simulink model "generic_IVS"  (R2024a)
settings: Solver=FixedStepDiscrete  StartTime=0.0  StopTime=inf  FixedStep=0.001  RelTol=1e-3
undefined symbols (not defined in the file): do_waypoints_tail_shifted_2, pathXY, route1_waypoint, route1_waypoint_raw, route2_waypoint, route2_waypoint_raw, route3_waypoint, route3_waypoint_raw, waypoints2
libraries: CarMaker4SL x431, slpidlib x19, dspsigops x3, simulink x1
(part 7 of 15)

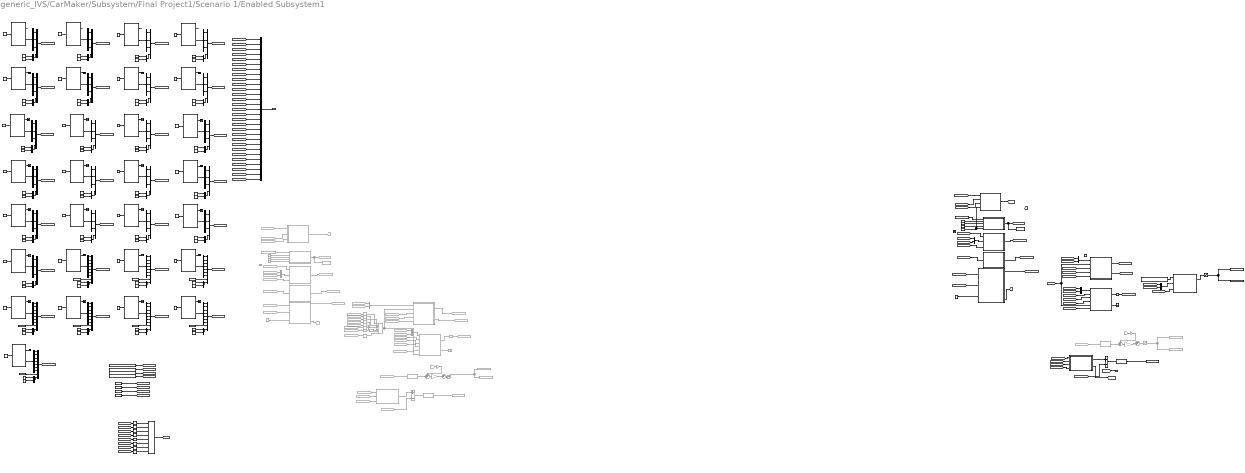
== system generic_IVS/CarMaker/Subsystem/Final Project1/Scenario 1/Enabled Subsystem1 ==
  note: Traffic Size
      | Length: 4.47
      | Width: 1.97
      | Height: 1.12
  note: 주행 개인
  note: Traffic Size
      | Length: 4.47
      | Width: 1.97
      | Height: 1.12
  note: Traffic Size
      | Length: 4.47
      | Width: 1.97
      | Height: 1.12
  note: Traffic Size
      | Length: 4.47
      | Width: 1.97
      | Height: 1.12
  note: Traffic Size
      | Length: 4.47
      | Width: 1.97
      | Height: 1.12
  note: Traffic Size
      | Length: 4.47
      | Width: 1.97
      | Height: 1.12
  note: Traffic Size
      | Length: 4.47
      | Width: 1.97
      | Height: 1.12
  note: Traffic Size
      | Length: 4.47
      | Width: 1.97
      | Height: 1.12
  note: 파킹 개인
  note: Traffic Size
      | Length: 4.47
      | Width: 1.97
      | Height: 1.12
  note: Traffic Size
      | Length: 4.47
      | Width: 1.97
      | Height: 1.12
  note: Traffic Size
      | Length: 4.47
      | Width: 1.97
      | Height: 1.12
  note: Traffic Size
      | Length: 4.47
      | Width: 1.97
      | Height: 1.12
  note: Traffic Size
      | Length: 4.47
      | Width: 1.97
      | Height: 1.12
  note: Traffic Size
      | Length: 4.47
      | Width: 1.97
      | Height: 1.12
  note: Traffic Size
      | Length: 4.47
      | Width: 1.97
      | Height: 1.12
  note: Traffic Size
      | Length: 4.47
      | Width: 1.97
      | Height: 1.12
  note: Traffic Size
      | Length: 4.47
      | Width: 1.97
      | Height: 1.12
  note: Traffic Size
      | Length: 4.47
      | Width: 1.97
      | Height: 1.12
  note: Traffic Size
      | Length: 4.47
      | Width: 1.97
      | Height: 1.12
  note: Traffic Size
      | Length: 4.47
      | Width: 1.97
      | Height: 1.12
  note: Traffic Size
      | Length: 4.47
      | Width: 1.97
      | Height: 1.12
  note: Modify !!
  note: Traffic Size
      | Length: 4.47
      | Width: 1.97
      | Height: 1.12
  note: Traffic Size
      | Length: 4.47
      | Width: 1.97
      | Height: 1.12
  note: Traffic Size
      | Length: 4.47
      | Width: 1.97
      | Height: 1.12
  note: Traffic Size
      | Length: 4.47
      | Width: 1.97
      | Height: 1.12
  note: Traffic Size
      | Length: 4.47
      | Width: 1.97
      | Height: 1.12
  note: Traffic Size
      | Length: 4.47
      | Width: 1.97
      | Height: 1.12
  note: 0: 파킹 경로, 1 주행, 2 파킹
  note: Traffic Size
      | Length: 4.47
      | Width: 1.97
      | Height: 1.12
  note: Average Filter
  note: Traffic Size
      | Length: 4.47
      | Width: 1.97
      | Height: 1.12
  note: Average Filter
  note: 0: 파킹 경로, 1 주행, 2 파킹
  note: Modify !!
  Enable : EnablePort
  Add : Sum  Inputs=+-
  Add1 : Sum  Commented=on  Inputs=+-
  Bus Selector{3..19,22,28..30} (21 alike) : BusSelector  OutputSignals=t_0 x,t_0 y,r_zyx z
  Bus Selector{20..21,23..27,31} (8 alike) : BusSelector  OutputSignals=t_0 x,t_0 y,v_0 x,v_0 y,a_0 x,a_0 y,r_zyx z
  Constant : Constant  Value=waypoints2
  Constant1 : Constant  Commented=on  Value=1565
  Constant10 : Constant  Commented=on
  Constant11 : Constant
  Constant110 : Constant  Value=do_waypoints_tail_shifted_2
  Constant111 : Constant  Value=1565
  Constant114 : Constant  Value=do_waypoints_tail_shifted_2
  Constant115 : Constant  Value=942
  Constant116 : Constant  Value=0
  Constant117 : Constant  Value=0
  Constant12 : Constant  Value=5
  Constant{13,16,19,21..22,26,29,32,35,39,42,46,48,52,55..56,59,61,65,69,72,74,79,82,85,87..88,92,96} (29 alike) : Constant  Value=4.47
  Constant{14,17,23..24,27,30,33,36..37,40,43,49..50,53,57,62..63,66..67,70,75..76,80,83,89..90,93..94,97} (29 alike) : Constant  Value=1.97
  Constant15 : Constant  Value=7
  Constant18 : Constant  Value=8
  Constant2 : Constant  Commented=on  Value=do_waypoints_tail_shifted_2
  Constant20 : Constant  Value=4
  Constant25 : Constant  Value=10
  Constant28 : Constant  Value=11
  Constant3 : Constant  Commented=on  Value=942
  Constant31 : Constant  Value=12
  Constant34 : Constant  Value=9
  Constant38 : Constant  Value=14
  Constant4 : Constant  Commented=on  Value=0
  Constant41 : Constant  Value=15
  Constant44 : Constant  Value=2
  Constant45 : Constant  Value=16
  Constant47 : Constant  Value=13
  Constant5 : Constant  Commented=on  Value=0
  Constant51 : Constant  Value=18
  Constant54 : Constant  Value=19
  Constant58 : Constant  Value=6
  Constant6 : Constant  Value=route1_waypoint_raw
  Constant60 : Constant  Value=17
  Constant64 : Constant  Value=21
  Constant68 : Constant  Value=22
  Constant7 : Constant
  Constant71 : Constant  Value=23
  Constant73 : Constant  Value=20
  Constant77 : Constant  Value=3
  Constant78 : Constant  Value=25
  Constant8 : Constant  Value=route2_waypoint_raw
  Constant81 : Constant  Value=26
  Constant84 : Constant  Value=27
  Constant86 : Constant  Value=24
  Constant9 : Constant  Value=route3_waypoint_raw
  Constant91 : Constant  Value=0
  Constant95 : Constant  Value=28
  From{49,53,87,90,100} (5 alike) : From  Commented=on  GotoTag=Ego_Gloabl_Y
  From101 : From  Commented=on  GotoTag=Ego_Velocity
  From102 : From  Commented=on  GotoTag=LateralError
  From34 : From  Commented=on  GotoTag=Global_Waypoints4
  From35 : From  Commented=on  GotoTag=Ego_Yaw
  From36 : From  Commented=on  GotoTag=Global_Waypoints1
  From37 : From  Commented=on  GotoTag=Global_Waypoints2
  From38 : From  Commented=on  GotoTag=Global_Waypoints3
  From{48,50,85,89,97} (5 alike) : From  Commented=on  GotoTag=Ego_Global_X
  From51 : From  Commented=on  GotoTag=Traffic_Info_21
  From52 : From  Commented=on  GotoTag=Traffic_Info_22
  From56 : From  Commented=on  GotoTag=Traffic_Info_23
  From58 : From  Commented=on  GotoTag=delta
  From63 : From  Commented=on  GotoTag=Traffic_Info_24
  From64 : From  Commented=on  GotoTag=Traffic_Info_25
  From65 : From  Commented=on  GotoTag=Traffic_Info_26
  From66 : From  Commented=on  GotoTag=Ego_Velocity
  From67 : From  Commented=on  GotoTag=Target_speed2
  From71 : From  Commented=on  GotoTag=Traffic_Info_27
  From72 : From  Commented=on  GotoTag=delta
  From86 : From  Commented=on  GotoTag=Local_Points
  From88 : From  Commented=on  GotoTag=New_Waypoint
  From9 : From  Commented=on  GotoTag=LateralError
  From91 : From  Commented=on  GotoTag=Ego_Yaw
  From92 : From  Commented=on  GotoTag=ego_lane_idx
  From93 : From  Commented=on  GotoTag=traffic_lane_idx
  From96 : From  Commented=on  GotoTag=Coefficients
  From98 : From  Commented=on  GotoTag=Ego_Velocity
  From99 : From  Commented=on  GotoTag=Traffic_Info_28
  Gain : Gain  Commented=on  Gain=pi/180
  Gain1 : Gain  Commented=on  Gain=3
  Gain2 : Gain  Commented=on  Gain=pi/180
  Gain3 : Gain  Commented=on  Gain=3
  Goto10 : Goto  Commented=on  GotoTag=flag
  Goto11 : Goto  Commented=on  GotoTag=New_Waypoint
  Goto42 : Goto  Commented=on  GotoTag=traffic_lane_idx
  Goto43 : Goto  Commented=on  GotoTag=ego_lane_idx
  Goto45 : Goto  Commented=on  GotoTag=Target_speed2
  Goto6 : Goto  Commented=on  GotoTag=delta
  Goto7 : Goto  Commented=on  GotoTag=Local_Points
  Goto8 : Goto  Commented=on  GotoTag=Coefficients
  Goto9 : Goto  Commented=on  GotoTag=LateralError
  Ground : Ground
  Ground1 : Ground  Commented=on
  MATLAB Function : MATLAB Function  TreatAsAtomicUnit=on
  MATLAB Function1 : MATLAB Function  TreatAsAtomicUnit=on
  MATLAB Function10 : MATLAB Function  Commented=on  TreatAsAtomicUnit=on
  MATLAB Function11 : MATLAB Function  Commented=on  TreatAsAtomicUnit=on
  MATLAB Function12 : MATLAB Function  TreatAsAtomicUnit=on
  MATLAB Function2 : MATLAB Function  Commented=on  TreatAsAtomicUnit=on
  MATLAB Function3 : MATLAB Function  TreatAsAtomicUnit=on
  MATLAB Function4 : MATLAB Function  TreatAsAtomicUnit=on
  "MATLAB Function4 " : MATLAB Function  TreatAsAtomicUnit=on
  MATLAB Function4 1 : MATLAB Function  TreatAsAtomicUnit=on
  MATLAB Function4 2 : MATLAB Function  Commented=on  TreatAsAtomicUnit=on
  MATLAB Function4 3 : MATLAB Function  Commented=on  TreatAsAtomicUnit=on
  MATLAB Function5 : MATLAB Function  TreatAsAtomicUnit=on
  MATLAB Function6 : MATLAB Function  TreatAsAtomicUnit=on
  MATLAB Function7 : MATLAB Function  Commented=on  TreatAsAtomicUnit=on
  MATLAB Function8 : MATLAB Function  Commented=on  TreatAsAtomicUnit=on
  MATLAB Function9 : MATLAB Function  Commented=on  TreatAsAtomicUnit=on
  Matrix Concatenate : Concatenate  Commented=on  NumInputs=8  Mode=Multidimensional array
  Matrix Concatenate2 : Concatenate  NumInputs=8  Mode=Multidimensional array
  Mux{,3..4,7..8,11,13,15,17,19,21,23,25,27,29,31,33,35,37,39,41,43,45,47,49,51,53,55..56,58,61,63,65} (33 alike) : Mux  Inputs=2
  Mux{1,5,9..10,12,14,16,18,20,22,24,26,28,30,32,34,36,38,46,57,60} (21 alike) : Mux
  Mux2 : Mux  Commented=on  Inputs=2
  Mux{40,42,44,48,50,52,54,64} (8 alike) : Mux  Inputs=9
  Mux59 : Mux  Inputs=29
  Mux6 : Mux  Commented=on  Inputs=2
  Mux62 : Mux  Commented=on  Inputs=2
  PID Controller1 : slpidlib/PID Controller  Controller=PID  Form=Ideal  TimeDomain=Discrete-time  UseExternalTs=off  SampleTime=-1  IntegratorMethod=Forward Euler  FilterMethod=Forward Euler  ControllerParametersSource=internal  P=3  I=0  UseKiTs=off  D=0.1  UseExternalDerivativeSource=off  N=1000  UseFilter=off  TunerSelectOption=Transfer Function Based (PID Tuner App)  InitialConditionSource=internal  InitialConditionForIntegrator=0  InitialConditionForFilter=0  DifferentiatorICPrevScaledInput=0  ExternalReset=none  TrackingMode=off  Kt=1  LimitOutput=off  SatLimitsSource=internal  UpperSaturationLimit=1  LowerSaturationLimit=-1  LinearizeAsGain=on  AntiWindupMode=back-calculation  Kb=1  LimitIntegrator=off  UpperIntegratorSaturationLimit=0.7  LowerIntegratorSaturationLimit=-0.7  POutMin=[]  POutMax=[]  IOutMin=[]  IOutMax=[]  DOutMin=[]  DOutMax=[]  NOutMin=[]  NOutMax=[]  SumOutMin=[]  SumOutMax=[]  SaturationOutMin=[]  SaturationOutMax=[]  PParamMin=[]  PParamMax=[]  IParamMin=[]  IParamMax=[]  DParamMin=[]  DParamMax=[]  NParamMin=[]  NParamMax=[]  KbParamMin=[]  KbParamMax=[]  KtParamMin=[]  KtParamMax=[]  KbOutMin=[]  KbOutMax=[]  KtOutMin=[]  KtOutMax=[]  IntegratorOutMin=[]  IntegratorOutMax=[]  FilterOutMin=[]  FilterOutMax=[]  SumI1OutMin=[]  SumI1OutMax=[]  SumI2OutMin=[]  SumI2OutMax=[]  SumI3OutMin=[]  SumI3OutMax=[]  SumI4OutMin=[]  SumI4OutMax=[]  SumDOutMin=[]  SumDOutMax=[]  DifferentiatorOutMin=[]  DifferentiatorOutMax=[]  FilterDiffOutCoefMin=[]  FilterDiffOutCoefMax=[]  ReciprocalOutMin=[]  ReciprocalOutMax=[]  SumDenOutMin=[]  SumDenOutMax=[]  SumNumOutMin=[]  SumNumOutMax=[]  DivideOutMin=[]  DivideOutMax=[]  UdiffTsProdOutMin=[]  UdiffTsProdOutMax=[]  NTsProdOutMin=[]  NTsProdOutMax=[]  UintegralTsProdOutMin=[]  UintegralTsProdOutMax=[]  UngainTsProdOutMin=[]  UngainTsProdOutMax=[]  ClampingZeroOutDataTypeStr=Inherit: Inherit via back propagation  ClampingZeroOutMin=[]  ClampingZeroOutMax=[]  FilterDenConstantOutDataTypeStr=Inherit: Inherit via back propagation  FilterDenConstantOutMin=[]  FilterDenConstantOutMax=[]  PCopyOutDataTypeStr=Inherit: Inherit via back propagation  PCopyOutMin=[]  PCopyOutMax=[]  NCopyOutDataTypeStr=Inherit: Inherit via back propagation  NCopyOutMin=[]  NCopyOutMax=[]  IntegratorContinuousStateAttributes=''  IntegratorStateMustResolveToSignalObject=off  IntegratorRTWStateStorageClass=Auto  FilterContinuousStateAttributes=''  FilterStateMustResolveToSignalObject=off  FilterRTWStateStorageClass=Auto  ParallelPVariant=Passthrough  IdealPVariant=InternalParameters  IVariant=InternalParameters  DVariant=InternalParameters  IntegratorVariant=Discrete  SatVariant=Disabled  AWVariant=Passthrough  PCopyVariant=Disabled  TRVariant=Disabled  FdbkBlocksVariant=Forward  IdealPFdbkVariant=Disabled  SatFdbkVariant=Disabled  DerivativeFilterVariant=Differentiator  NVariant=Passthrough  NCopyVariant=Disabled_SignalSpec  FilterICVariant=InternalICsDifferentiator  IntegratorICVariant=InternalICs  ExternalResetVariant=Disabled  TRSumVariant=Passthrough  SumFdbkVariant=Disabled  SumVariant=Sum_PID  TsampFilterVariant=InternalTs  TsampNgainVariant=Passthrough  TsampIntegralVariant=Disabled_SignalSpec  ExternalSaturationOutDataTypeStr=Inherit: Same as second input  DerivativeSourceVariant=ErrorSignal
  PID Controller2 : slpidlib/PID Controller  Commented=on  Controller=PID  Form=Ideal  TimeDomain=Discrete-time  UseExternalTs=off  SampleTime=-1  IntegratorMethod=Forward Euler  FilterMethod=Forward Euler  ControllerParametersSource=internal  P=3  I=0  UseKiTs=off  D=0.1  UseExternalDerivativeSource=off  N=1000  UseFilter=off  TunerSelectOption=Transfer Function Based (PID Tuner App)  InitialConditionSource=internal  InitialConditionForIntegrator=0  InitialConditionForFilter=0  DifferentiatorICPrevScaledInput=0  ExternalReset=none  TrackingMode=off  Kt=1  LimitOutput=off  SatLimitsSource=internal  UpperSaturationLimit=1  LowerSaturationLimit=-1  LinearizeAsGain=on  AntiWindupMode=back-calculation  Kb=1  LimitIntegrator=off  UpperIntegratorSaturationLimit=0.7  LowerIntegratorSaturationLimit=-0.7  POutMin=[]  POutMax=[]  IOutMin=[]  IOutMax=[]  DOutMin=[]  DOutMax=[]  NOutMin=[]  NOutMax=[]  SumOutMin=[]  SumOutMax=[]  SaturationOutMin=[]  SaturationOutMax=[]  PParamMin=[]  PParamMax=[]  IParamMin=[]  IParamMax=[]  DParamMin=[]  DParamMax=[]  NParamMin=[]  NParamMax=[]  KbParamMin=[]  KbParamMax=[]  KtParamMin=[]  KtParamMax=[]  KbOutMin=[]  KbOutMax=[]  KtOutMin=[]  KtOutMax=[]  IntegratorOutMin=[]  IntegratorOutMax=[]  FilterOutMin=[]  FilterOutMax=[]  SumI1OutMin=[]  SumI1OutMax=[]  SumI2OutMin=[]  SumI2OutMax=[]  SumI3OutMin=[]  SumI3OutMax=[]  SumI4OutMin=[]  SumI4OutMax=[]  SumDOutMin=[]  SumDOutMax=[]  DifferentiatorOutMin=[]  DifferentiatorOutMax=[]  FilterDiffOutCoefMin=[]  FilterDiffOutCoefMax=[]  ReciprocalOutMin=[]  ReciprocalOutMax=[]  SumDenOutMin=[]  SumDenOutMax=[]  SumNumOutMin=[]  SumNumOutMax=[]  DivideOutMin=[]  DivideOutMax=[]  UdiffTsProdOutMin=[]  UdiffTsProdOutMax=[]  NTsProdOutMin=[]  NTsProdOutMax=[]  UintegralTsProdOutMin=[]  UintegralTsProdOutMax=[]  UngainTsProdOutMin=[]  UngainTsProdOutMax=[]  ClampingZeroOutDataTypeStr=Inherit: Inherit via back propagation  ClampingZeroOutMin=[]  ClampingZeroOutMax=[]  FilterDenConstantOutDataTypeStr=Inherit: Inherit via back propagation  FilterDenConstantOutMin=[]  FilterDenConstantOutMax=[]  PCopyOutDataTypeStr=Inherit: Inherit via back propagation  PCopyOutMin=[]  PCopyOutMax=[]  NCopyOutDataTypeStr=Inherit: Inherit via back propagation  NCopyOutMin=[]  NCopyOutMax=[]  IntegratorContinuousStateAttributes=''  IntegratorStateMustResolveToSignalObject=off  IntegratorRTWStateStorageClass=Auto  FilterContinuousStateAttributes=''  FilterStateMustResolveToSignalObject=off  FilterRTWStateStorageClass=Auto  ParallelPVariant=Passthrough  IdealPVariant=InternalParameters  IVariant=InternalParameters  DVariant=InternalParameters  IntegratorVariant=Discrete  SatVariant=Disabled  AWVariant=Passthrough  PCopyVariant=Disabled  TRVariant=Disabled  FdbkBlocksVariant=Forward  IdealPFdbkVariant=Disabled  SatFdbkVariant=Disabled  DerivativeFilterVariant=Differentiator  NVariant=Passthrough  NCopyVariant=Disabled_SignalSpec  FilterICVariant=InternalICsDifferentiator  IntegratorICVariant=InternalICs  ExternalResetVariant=Disabled  TRSumVariant=Passthrough  SumFdbkVariant=Disabled  SumVariant=Sum_PID  TsampFilterVariant=InternalTs  TsampNgainVariant=Passthrough  TsampIntegralVariant=Disabled_SignalSpec  ExternalSaturationOutDataTypeStr=Inherit: Same as second input  DerivativeSourceVariant=ErrorSignal
  PID for parking : slpidlib/PID Controller  Commented=on  Controller=PID  Form=Ideal  TimeDomain=Discrete-time  UseExternalTs=off  SampleTime=-1  IntegratorMethod=Forward Euler  FilterMethod=Forward Euler  ControllerParametersSource=internal  P=5  I=0.4  UseKiTs=off  D=3  UseExternalDerivativeSource=off  N=1000  UseFilter=off  TunerSelectOption=Transfer Function Based (PID Tuner App)  InitialConditionSource=internal  InitialConditionForIntegrator=0  InitialConditionForFilter=0  DifferentiatorICPrevScaledInput=0  ExternalReset=none  TrackingMode=off  Kt=1  LimitOutput=off  SatLimitsSource=internal  UpperSaturationLimit=1  LowerSaturationLimit=-1  LinearizeAsGain=on  AntiWindupMode=back-calculation  Kb=1  LimitIntegrator=on  UpperIntegratorSaturationLimit=1  LowerIntegratorSaturationLimit=-1  POutMin=[]  POutMax=[]  IOutMin=[]  IOutMax=[]  DOutMin=[]  DOutMax=[]  NOutMin=[]  NOutMax=[]  SumOutMin=[]  SumOutMax=[]  SaturationOutMin=[]  SaturationOutMax=[]  PParamMin=[]  PParamMax=[]  IParamMin=[]  IParamMax=[]  DParamMin=[]  DParamMax=[]  NParamMin=[]  NParamMax=[]  KbParamMin=[]  KbParamMax=[]  KtParamMin=[]  KtParamMax=[]  KbOutMin=[]  KbOutMax=[]  KtOutMin=[]  KtOutMax=[]  IntegratorOutMin=[]  IntegratorOutMax=[]  FilterOutMin=[]  FilterOutMax=[]  SumI1OutMin=[]  SumI1OutMax=[]  SumI2OutMin=[]  SumI2OutMax=[]  SumI3OutMin=[]  SumI3OutMax=[]  SumI4OutMin=[]  SumI4OutMax=[]  SumDOutMin=[]  SumDOutMax=[]  DifferentiatorOutMin=[]  DifferentiatorOutMax=[]  FilterDiffOutCoefMin=[]  FilterDiffOutCoefMax=[]  ReciprocalOutMin=[]  ReciprocalOutMax=[]  SumDenOutMin=[]  SumDenOutMax=[]  SumNumOutMin=[]  SumNumOutMax=[]  DivideOutMin=[]  DivideOutMax=[]  UdiffTsProdOutMin=[]  UdiffTsProdOutMax=[]  NTsProdOutMin=[]  NTsProdOutMax=[]  UintegralTsProdOutMin=[]  UintegralTsProdOutMax=[]  UngainTsProdOutMin=[]  UngainTsProdOutMax=[]  ClampingZeroOutDataTypeStr=Inherit: Inherit via back propagation  ClampingZeroOutMin=[]  ClampingZeroOutMax=[]  FilterDenConstantOutDataTypeStr=Inherit: Inherit via back propagation  FilterDenConstantOutMin=[]  FilterDenConstantOutMax=[]  PCopyOutDataTypeStr=Inherit: Inherit via back propagation  PCopyOutMin=[]  PCopyOutMax=[]  NCopyOutDataTypeStr=Inherit: Inherit via back propagation  NCopyOutMin=[]  NCopyOutMax=[]  IntegratorContinuousStateAttributes=''  IntegratorStateMustResolveToSignalObject=off  IntegratorRTWStateStorageClass=Auto  FilterContinuousStateAttributes=''  FilterStateMustResolveToSignalObject=off  FilterRTWStateStorageClass=Auto  ParallelPVariant=Passthrough  IdealPVariant=InternalParameters  IVariant=InternalParameters  DVariant=InternalParameters  IntegratorVariant=Discrete  SatVariant=Disabled  AWVariant=Passthrough  PCopyVariant=Disabled  TRVariant=Disabled  FdbkBlocksVariant=Forward  IdealPFdbkVariant=Disabled  SatFdbkVariant=Disabled  DerivativeFilterVariant=Differentiator  NVariant=Passthrough  NCopyVariant=Disabled_SignalSpec  FilterICVariant=InternalICsDifferentiator  IntegratorICVariant=InternalICs  ExternalResetVariant=Disabled  TRSumVariant=Passthrough  SumFdbkVariant=Disabled  SumVariant=Sum_PID  TsampFilterVariant=InternalTs  TsampNgainVariant=Passthrough  TsampIntegralVariant=Disabled_SignalSpec  ExternalSaturationOutDataTypeStr=Inherit: Same as second input  DerivativeSourceVariant=ErrorSignal
  PID for parking1 : slpidlib/PID Controller  Commented=on  Controller=PID  Form=Ideal  TimeDomain=Discrete-time  UseExternalTs=off  SampleTime=-1  IntegratorMethod=Forward Euler  FilterMethod=Forward Euler  ControllerParametersSource=internal  P=5  I=0.4  UseKiTs=off  D=3  UseExternalDerivativeSource=off  N=1000  UseFilter=off  TunerSelectOption=Transfer Function Based (PID Tuner App)  InitialConditionSource=internal  InitialConditionForIntegrator=0  InitialConditionForFilter=0  DifferentiatorICPrevScaledInput=0  ExternalReset=none  TrackingMode=off  Kt=1  LimitOutput=off  SatLimitsSource=internal  UpperSaturationLimit=1  LowerSaturationLimit=-1  LinearizeAsGain=on  AntiWindupMode=back-calculation  Kb=1  LimitIntegrator=on  UpperIntegratorSaturationLimit=1  LowerIntegratorSaturationLimit=-1  POutMin=[]  POutMax=[]  IOutMin=[]  IOutMax=[]  DOutMin=[]  DOutMax=[]  NOutMin=[]  NOutMax=[]  SumOutMin=[]  SumOutMax=[]  SaturationOutMin=[]  SaturationOutMax=[]  PParamMin=[]  PParamMax=[]  IParamMin=[]  IParamMax=[]  DParamMin=[]  DParamMax=[]  NParamMin=[]  NParamMax=[]  KbParamMin=[]  KbParamMax=[]  KtParamMin=[]  KtParamMax=[]  KbOutMin=[]  KbOutMax=[]  KtOutMin=[]  KtOutMax=[]  IntegratorOutMin=[]  IntegratorOutMax=[]  FilterOutMin=[]  FilterOutMax=[]  SumI1OutMin=[]  SumI1OutMax=[]  SumI2OutMin=[]  SumI2OutMax=[]  SumI3OutMin=[]  SumI3OutMax=[]  SumI4OutMin=[]  SumI4OutMax=[]  SumDOutMin=[]  SumDOutMax=[]  DifferentiatorOutMin=[]  DifferentiatorOutMax=[]  FilterDiffOutCoefMin=[]  FilterDiffOutCoefMax=[]  ReciprocalOutMin=[]  ReciprocalOutMax=[]  SumDenOutMin=[]  SumDenOutMax=[]  SumNumOutMin=[]  SumNumOutMax=[]  DivideOutMin=[]  DivideOutMax=[]  UdiffTsProdOutMin=[]  UdiffTsProdOutMax=[]  NTsProdOutMin=[]  NTsProdOutMax=[]  UintegralTsProdOutMin=[]  UintegralTsProdOutMax=[]  UngainTsProdOutMin=[]  UngainTsProdOutMax=[]  ClampingZeroOutDataTypeStr=Inherit: Inherit via back propagation  ClampingZeroOutMin=[]  ClampingZeroOutMax=[]  FilterDenConstantOutDataTypeStr=Inherit: Inherit via back propagation  FilterDenConstantOutMin=[]  FilterDenConstantOutMax=[]  PCopyOutDataTypeStr=Inherit: Inherit via back propagation  PCopyOutMin=[]  PCopyOutMax=[]  NCopyOutDataTypeStr=Inherit: Inherit via back propagation  NCopyOutMin=[]  NCopyOutMax=[]  IntegratorContinuousStateAttributes=''  IntegratorStateMustResolveToSignalObject=off  IntegratorRTWStateStorageClass=Auto  FilterContinuousStateAttributes=''  FilterStateMustResolveToSignalObject=off  FilterRTWStateStorageClass=Auto  ParallelPVariant=Passthrough  IdealPVariant=InternalParameters  IVariant=InternalParameters  DVariant=InternalParameters  IntegratorVariant=Discrete  SatVariant=Disabled  AWVariant=Passthrough  PCopyVariant=Disabled  TRVariant=Disabled  FdbkBlocksVariant=Forward  IdealPFdbkVariant=Disabled  SatFdbkVariant=Disabled  DerivativeFilterVariant=Differentiator  NVariant=Passthrough  NCopyVariant=Disabled_SignalSpec  FilterICVariant=InternalICsDifferentiator  IntegratorICVariant=InternalICs  ExternalResetVariant=Disabled  TRSumVariant=Passthrough  SumFdbkVariant=Disabled  SumVariant=Sum_PID  TsampFilterVariant=InternalTs  TsampNgainVariant=Passthrough  TsampIntegralVariant=Disabled_SignalSpec  ExternalSaturationOutDataTypeStr=Inherit: Same as second input  DerivativeSourceVariant=ErrorSignal
  Rate Limiter : RateLimiter  Commented=on  RisingSlewLimit=1.1  FallingSlewLimit=-3.0  SampleTimeMode=inherited  InitialCondition=13.0
  Rate Limiter1 : RateLimiter  RisingSlewLimit=1.1  FallingSlewLimit=-3.0  SampleTimeMode=inherited  InitialCondition=13.0
  Read CM Dict22 : CarMaker4SL/Read CM Dict  xname=Traffic.T21.rzv  xsync=off  xstime=Inherited
  Read CM Dict23 : CarMaker4SL/Read CM Dict  xname=Traffic.T22.rzv  xsync=off  xstime=Inherited
  Read CM Dict24 : CarMaker4SL/Read CM Dict  xname=Traffic.T23.rzv  xsync=off  xstime=Inherited
  Read CM Dict25 : CarMaker4SL/Read CM Dict  xname=Traffic.T24.rzv  xsync=off  xstime=Inherited
  Read CM Dict26 : CarMaker4SL/Read CM Dict  xname=Traffic.T25.rzv  xsync=off  xstime=Inherited
  Read CM Dict27 : CarMaker4SL/Read CM Dict  xname=Traffic.T26.rzv  xsync=off  xstime=Inherited
  Read CM Dict28 : CarMaker4SL/Read CM Dict  xname=Traffic.T27.rzv  xsync=off  xstime=Inherited
  Read CM Dict29 : CarMaker4SL/Read CM Dict  xname=Traffic.T28.rzv  xsync=off  xstime=Inherited
  Read CM Dict5 : CarMaker4SL/Read CM Dict  xname=Car.Fr1.tx  xsync=off  xstime=Inherited
  Read CM Dict6 : CarMaker4SL/Read CM Dict  xname=Car.Fr1.ty  xsync=off  xstime=Inherited
  Read CM Dict7 : CarMaker4SL/Read CM Dict  xname=Car.v  xsync=off  xstime=Inherited
  Read CM Dict8 : CarMaker4SL/Read CM Dict  xname=Car.Fr1.rz  xsync=off  xstime=Inherited
  Saturation1 : Saturate  Commented=on  UpperLimit=2  LowerLimit=-2
  Saturation2 : Saturate  Commented=on  UpperLimit=2  LowerLimit=-2
  Saturation3 : Saturate  UpperLimit=2  LowerLimit=-2
  Scope1 : Scope  Commented=on
  Scope8 : Scope
  Sum{,1..3} (4 alike) : Sum  Commented=on  Inputs=++|
  Terminator{7..31} (25 alike) : Terminator
  To Workspace : ToWorkspace  VariableName=waypoint_test1  SaveFormat=Timeseries  SampleTime=-1
  To Workspace1 : ToWorkspace  Commented=on  VariableName=waypoint_test  SaveFormat=Timeseries  SampleTime=-1
  Traffic Object10 : CarMaker4SL/Traffic Object  xname=T11  ximode=Traffic Id  xstime=Inherited
      settings: SourceProductName=CarMaker4SL
  Traffic Object11 : CarMaker4SL/Traffic Object  xname=T12  ximode=Traffic Id  xstime=Inherited
      settings: SourceProductName=CarMaker4SL
  Traffic Object12 : CarMaker4SL/Traffic Object  xname=T13  ximode=Traffic Id  xstime=Inherited
      settings: SourceProductName=CarMaker4SL
  Traffic Object13 : CarMaker4SL/Traffic Object  xname=T14  ximode=Traffic Id  xstime=Inherited
      settings: SourceProductName=CarMaker4SL
  Traffic Object14 : CarMaker4SL/Traffic Object  xname=T15  ximode=Traffic Id  xstime=Inherited
      settings: SourceProductName=CarMaker4SL
  Traffic Object15 : CarMaker4SL/Traffic Object  xname=T16  ximode=Traffic Id  xstime=Inherited
      settings: SourceProductName=CarMaker4SL
  Traffic Object16 : CarMaker4SL/Traffic Object  xname=T17  ximode=Traffic Id  xstime=Inherited
      settings: SourceProductName=CarMaker4SL
  Traffic Object17 : CarMaker4SL/Traffic Object  xname=T18  ximode=Traffic Id  xstime=Inherited
      settings: SourceProductName=CarMaker4SL
  Traffic Object18 : CarMaker4SL/Traffic Object  xname=T19  ximode=Traffic Id  xstime=Inherited
      settings: SourceProductName=CarMaker4SL
  Traffic Object19 : CarMaker4SL/Traffic Object  xname=T06  ximode=Traffic Id  xstime=Inherited
      settings: SourceProductName=CarMaker4SL
  Traffic Object20 : CarMaker4SL/Traffic Object  xname=T20  ximode=Traffic Id  xstime=Inherited
      settings: SourceProductName=CarMaker4SL
  Traffic Object21 : CarMaker4SL/Traffic Object  xname=T21  ximode=Traffic Id  xstime=Inherited
      settings: SourceProductName=CarMaker4SL
  Traffic Object22 : CarMaker4SL/Traffic Object  xname=T22  ximode=Traffic Id  xstime=Inherited
      settings: SourceProductName=CarMaker4SL
  Traffic Object23 : CarMaker4SL/Traffic Object  xname=T23  ximode=Traffic Id  xstime=Inherited
      settings: SourceProductName=CarMaker4SL
  Traffic Object24 : CarMaker4SL/Traffic Object  xname=T24  ximode=Traffic Id  xstime=Inherited
      settings: SourceProductName=CarMaker4SL
  Traffic Object25 : CarMaker4SL/Traffic Object  xname=T25  ximode=Traffic Id  xstime=Inherited
      settings: SourceProductName=CarMaker4SL
  Traffic Object26 : CarMaker4SL/Traffic Object  xname=T26  ximode=Traffic Id  xstime=Inherited
      settings: SourceProductName=CarMaker4SL
  Traffic Object27 : CarMaker4SL/Traffic Object  xname=T27  ximode=Traffic Id  xstime=Inherited
      settings: SourceProductName=CarMaker4SL
  Traffic Object28 : CarMaker4SL/Traffic Object  xname=T28  ximode=Traffic Id  xstime=Inherited
      settings: SourceProductName=CarMaker4SL
  Traffic Object29 : CarMaker4SL/Traffic Object  xname=T08  ximode=Traffic Id  xstime=Inherited
      settings: SourceProductName=CarMaker4SL
  Traffic Object3 : CarMaker4SL/Traffic Object  xname=T00  ximode=Traffic Id  xstime=Inherited
      settings: SourceProductName=CarMaker4SL
  Traffic Object30 : CarMaker4SL/Traffic Object  xname=T09  ximode=Traffic Id  xstime=Inherited
      settings: SourceProductName=CarMaker4SL
  Traffic Object31 : CarMaker4SL/Traffic Object  xname=T10  ximode=Traffic Id  xstime=Inherited
      settings: SourceProductName=CarMaker4SL
  Traffic Object4 : CarMaker4SL/Traffic Object  xname=T01  ximode=Traffic Id  xstime=Inherited
      settings: SourceProductName=CarMaker4SL
  Traffic Object5 : CarMaker4SL/Traffic Object  xname=T02  ximode=Traffic Id  xstime=Inherited
      settings: SourceProductName=CarMaker4SL
  Traffic Object6 : CarMaker4SL/Traffic Object  xname=T03  ximode=Traffic Id  xstime=Inherited
      settings: SourceProductName=CarMaker4SL
  Traffic Object7 : CarMaker4SL/Traffic Object  xname=T04  ximode=Traffic Id  xstime=Inherited
      settings: SourceProductName=CarMaker4SL
  Traffic Object8 : CarMaker4SL/Traffic Object  xname=T05  ximode=Traffic Id  xstime=Inherited
      settings: SourceProductName=CarMaker4SL
  Traffic Object9 : CarMaker4SL/Traffic Object  xname=T07  ximode=Traffic Id  xstime=Inherited
      settings: SourceProductName=CarMaker4SL
  Transpose{,1..7} (8 alike) : Math  Commented=on  Operator=transpose
  Transpose{8..16} (9 alike) : Math  Operator=transpose
  Write CM Dict1 : CarMaker4SL/Write CM Dict  Commented=on  xname=Car.CFL.rz_ext  xsync=off
  Write CM Dict2 : CarMaker4SL/Write CM Dict  Commented=on  xname=Car.CFR.rz_ext  xsync=off
  Write CM Dict3 : CarMaker4SL/Write CM Dict  Commented=on  xname=Car.CFL.rz_ext  xsync=off
  Write CM Dict4 : CarMaker4SL/Write CM Dict  Commented=on  xname=Car.CFR.rz_ext  xsync=off
  Write CM Dict5 : CarMaker4SL/Write CM Dict  xname=AccelCtrl.DesiredAx  xsync=off
  Write CM Dict6 : CarMaker4SL/Write CM Dict  Commented=on  xname=AccelCtrl.DesiredAx  xsync=off
  Write CM Dict7 : CarMaker4SL/Write CM Dict  xname=Car.CFL.rz_ext  xsync=off
  Write CM Dict8 : CarMaker4SL/Write CM Dict  xname=Car.CFR.rz_ext  xsync=off
  Traffic_Info : Outport
  Output1 : Outport  Port=2
  wires:
  "MATLAB Function4 "/1(local_waypoints_) -> [Local_Points]
  [Traffic_Info_20] -> Mux59/21
  Constant37/1 -> Mux23/2
  [Traffic_Info_22] -> Transpose9/1
  Mux39/1 -> Mux38/4
  Constant23/1 -> Mux13/2
  Traffic Object16/2 -> Bus Selector18/1
  Bus Selector27/4 -> Mux52/4  "<v_0 y>"
  Bus Selector23/1 -> Mux44/1  "<t_0 x>"
  Bus Selector28/1 -> Mux16/1  "<t_0 x>"
  [Ego_Gloabl_Y] -> Mux7/2
  [Traffic_Info_22] -> Mux59/23
  Bus Selector20/3 -> Mux40/3  "<v_0 x>"
  Constant66/1 -> Mux8/2
  Bus Selector20/5 -> Mux40/5  "<a_0 x>"
  [Traffic_Info_15] -> Mux59/16
  Mux8/1 -> Mux5/4
  Mux41/1 -> Mux40/9
  Constant110/1 -> [Global_Waypoints4]
  Traffic Object8/1 -> Terminator8/1
  Traffic Object10/2 -> Bus Selector30/1
  [traffic_lane_idx] -> MATLAB Function5/6(traffic_lane_idx)
  Mux60/1 -> [Traffic_Info_00]
  Bus Selector23/4 -> Mux44/4  "<v_0 y>"
  Bus Selector28/3 -> Mux16/3  "<r_zyx z>"
  Mux17/1 -> Mux16/4
  Mux33/1 -> Mux32/4
  Mux19/1 -> Mux18/4
  Mux52/1 -> [Traffic_Info_27]
  Bus Selector19/1 -> Mux36/1  "<t_0 x>"
  Mux38/1 -> [Traffic_Info_17]
  Constant6/1 -> [Global_Waypoints1]
  Bus Selector21/5 -> Mux42/5  "<a_0 x>"
  Bus Selector22/3 -> Mux46/3  "<r_zyx z>"
  Mux11/1 -> Mux10/4
  [Traffic_Info_27] -> Transpose14/1
  Bus Selector30/1 -> Mux18/1  "<t_0 x>"
  Traffic Object3/2 -> Bus Selector29/1
  Constant53/1 -> Mux33/2
  Mux65/1 -> Mux64/9
  Mux23/1 -> Mux22/4
  Constant28/1 -> Traffic Object10/1
  Transpose13/1 -> Matrix Concatenate2/6
  Mux30/1 -> [Traffic_Info_13]
  Constant95/1 -> Traffic Object28/1
  Mux12/1 -> [Traffic_Info_08]
  Mux16/1 -> [Traffic_Info_10]
  Traffic Object28/1 -> Terminator28/1
  Constant38/1 -> Traffic Object13/1
  Constant35/1 -> Mux23/1
  Bus Selector29/2 -> Mux60/2  "<t_0 y>"
  Traffic Object9/2 -> Bus Selector7/1
  Traffic Object23/1 -> Terminator23/1
  [Ego_Global_X] -> Mux3/1
  Mux25/1 -> Mux24/4
  MATLAB Function4/1(poly_coeff) -> [Coefficients]
  [Traffic_Info_24] -> Mux59/25
  Mux7/1 -> MATLAB Function5/1(ego_pos)
  [Traffic_Info_01] -> Mux59/2
  Constant27/1 -> Mux17/2
  Read CM Dict22/1 -> Mux40/8
  Bus Selector12/3 -> Mux24/3  "<r_zyx z>"
  [Ego_Global_X] -> Mux7/1
  Constant52/1 -> Mux33/1
  Traffic Object16/1 -> Terminator16/1
  Bus Selector11/1 -> Mux20/1  "<t_0 x>"
  Constant81/1 -> Traffic Object26/1
  Constant87/1 -> Mux55/1
  [Traffic_Info_26] -> Mux59/27
  Mux44/1 -> [Traffic_Info_23]
  Constant29/1 -> Mux19/1
  [Traffic_Info_17] -> Mux59/18
  Bus Selector31/6 -> Mux64/6  "<a_0 y>"
  [Traffic_Info_19] -> Mux59/20
  Traffic Object18/2 -> Bus Selector17/1
  Mux31/1 -> Mux30/4
  Traffic Object14/1 -> Terminator14/1
  Traffic Object11/1 -> Terminator11/1
  Bus Selector31/1 -> Mux64/1  "<t_0 x>"
  Mux49/1 -> Mux48/9
  Bus Selector26/7 -> Mux54/7  "<r_zyx z>"
  Bus Selector21/6 -> Mux42/6  "<a_0 y>"
  [Traffic_Info_25] -> Mux59/26
  Traffic Object7/1 -> Terminator7/1
  Bus Selector26/4 -> Mux54/4  "<v_0 y>"
  Bus Selector9/2 -> Mux12/2  "<t_0 y>"
  Bus Selector12/2 -> Mux24/2  "<t_0 y>"
  Constant54/1 -> Traffic Object18/1
  Mux28/1 -> [Traffic_Info_16]
  Bus Selector18/3 -> Mux38/3  "<r_zyx z>"
  MATLAB Function1/1(target_speed_out) -> Add/1
  Read CM Dict26/1 -> Mux48/8
  Bus Selector24/1 -> Mux48/1  "<t_0 x>"
  Mux20/1 -> [Traffic_Info_12]
  Read CM Dict25/1 -> Mux54/8
  Bus Selector10/3 -> Mux22/3  "<r_zyx z>"
  Bus Selector5/2 -> Mux9/2  "<t_0 y>"
  Bus Selector13/3 -> Mux26/3  "<r_zyx z>"
  Traffic Object11/2 -> Bus Selector11/1
  Bus Selector30/2 -> Mux18/2  "<t_0 y>"
  Mux54/1 -> [Traffic_Info_24]
  Constant93/1 -> Mux56/2
  Mux13/1 -> Mux12/4
  Bus Selector26/6 -> Mux54/6  "<a_0 y>"
  Bus Selector30/3 -> Mux18/3  "<r_zyx z>"
  MATLAB Function5/1(target_speed) -> Rate Limiter1/1
  Read CM Dict29/1 -> Mux64/8
  Bus Selector24/7 -> Mux48/7  "<r_zyx z>"
  Bus Selector3/1 -> Mux1/1  "<t_0 x>"
  Constant21/1 -> Mux15/1
  Constant34/1 -> Traffic Object30/1
  [Ego_Velocity] -> MATLAB Function3/2(velocity)
  Bus Selector4/1 -> Mux5/1  "<t_0 x>"
  Bus Selector29/1 -> Mux60/1  "<t_0 x>"
  Read CM Dict28/1 -> Mux52/8
  Bus Selector27/2 -> Mux52/2  "<t_0 y>"
  Mux53/1 -> Mux52/9
  Constant89/1 -> Mux53/2
  Traffic Object20/2 -> Bus Selector22/1
  Bus Selector7/1 -> Mux10/1  "<t_0 x>"
  Bus Selector20/2 -> Mux40/2  "<t_0 y>"
  Read CM Dict6/1 -> [Ego_Gloabl_Y]
  [Traffic_Info_10] -> Mux59/11
  Traffic Object18/1 -> Terminator18/1
  Bus Selector3/2 -> Mux1/2  "<t_0 y>"
  Traffic Object24/1 -> Terminator24/1
  [Ego_Gloabl_Y] -> MATLAB Function1/2(u2)
  [Traffic_Info_24] -> Transpose11/1
  [Ego_Yaw] -> "MATLAB Function4 "/3(head)
  Constant90/1 -> Mux55/2
  Constant74/1 -> Mux47/1
  MATLAB Function3/6(kappa) -> [delta]
  Traffic Object25/1 -> Terminator25/1
  Constant40/1 -> Mux25/2
  Mux24/1 -> [Traffic_Info_14]
  Constant73/1 -> Traffic Object20/1
  [Traffic_Info_27] -> Mux59/28
  Traffic Object25/2 -> Bus Selector24/1
  [Coefficients] -> MATLAB Function3/1(poly_coeff)
  Constant46/1 -> Mux29/1
  Bus Selector4/3 -> Mux5/3  "<r_zyx z>"
  Constant18/1 -> Traffic Object29/1
  Traffic Object22/2 -> Bus Selector21/1
  Traffic Object27/1 -> Terminator27/1
  Traffic Object31/1 -> Terminator31/1
  Bus Selector14/1 -> Mux30/1  "<t_0 x>"
  Bus Selector27/5 -> Mux52/5  "<a_0 x>"
  Bus Selector16/2 -> Mux32/2  "<t_0 y>"
  Constant85/1 -> Mux53/1
  Constant86/1 -> Traffic Object24/1
  Bus Selector25/7 -> Mux50/7  "<r_zyx z>"
  [Traffic_Info_23] -> Mux59/24
  Traffic Object7/2 -> Bus Selector8/1
  Constant116/1 -> MATLAB Function/3(must1)
  [Traffic_Info_11] -> Mux59/12
  Read CM Dict5/1 -> [Ego_Global_X]
  Mux27/1 -> Mux26/4
  Bus Selector24/4 -> Mux48/4  "<v_0 y>"
  Mux29/1 -> Mux28/4
  Constant59/1 -> Mux37/1
  Mux48/1 -> [Traffic_Info_25]
  Bus Selector17/3 -> Mux34/3  "<r_zyx z>"
  Bus Selector18/1 -> Mux38/1  "<t_0 x>"
  [Traffic_Info_04] -> Mux59/5
  Mux61/1 -> Mux60/4
  Constant72/1 -> Mux45/1
  Constant115/1 -> MATLAB Function/2(startIdx)
  Bus Selector5/1 -> Mux9/1  "<t_0 x>"
  [Traffic_Info_09] -> Mux59/10
  Bus Selector27/3 -> Mux52/3  "<v_0 x>"
  Bus Selector19/3 -> Mux36/3  "<r_zyx z>"
  Bus Selector15/3 -> Mux28/3  "<r_zyx z>"
  Traffic Object19/2 -> Bus Selector19/1
  Transpose11/1 -> Matrix Concatenate2/4
  Mux21/1 -> Mux20/4
  MATLAB Function6/1(ego_lane_idx) -> [ego_lane_idx]
  Bus Selector26/5 -> Mux54/5  "<a_0 x>"
  Bus Selector12/1 -> Mux24/1  "<t_0 x>"
  Transpose14/1 -> Matrix Concatenate2/7
  Bus Selector31/4 -> Mux64/4  "<v_0 y>"
  Traffic Object23/2 -> Bus Selector23/1
  Mux43/1 -> Mux42/9
  Traffic Object21/1 -> Terminator21/1
  Bus Selector8/3 -> Mux14/3  "<r_zyx z>"
  Constant24/1 -> Mux15/2
  Mux56/1 -> Mux9/4
  Bus Selector18/2 -> Mux38/2  "<t_0 y>"
  PID Controller1/1 -> Write CM Dict5/1
  Mux32/1 -> [Traffic_Info_18]
  Bus Selector7/2 -> Mux10/2  "<t_0 y>"
  Traffic Object5/1 -> ?
  Constant75/1 -> Mux45/2
  [Traffic_Info_05] -> Mux59/6
  Read CM Dict7/1 -> [Ego_Velocity]
  Bus Selector25/2 -> Mux50/2  "<t_0 y>"
  Mux55/1 -> Mux54/9
  Bus Selector21/4 -> Mux42/4  "<v_0 y>"
  Bus Selector20/7 -> Mux40/7  "<r_zyx z>"
  Constant68/1 -> Traffic Object22/1
  Bus Selector23/7 -> Mux44/7  "<r_zyx z>"
  Traffic Object30/2 -> Bus Selector10/1
  Transpose9/1 -> Matrix Concatenate2/2
  Bus Selector6/2 -> Mux57/2  "<t_0 y>"
  Traffic Object12/2 -> Bus Selector14/1
  Constant61/1 -> Mux39/1
  Constant39/1 -> Mux25/1
  Traffic Object17/1 -> Terminator17/1
  [Traffic_Info_28] -> Transpose15/1
  Sum1/1 -> Gain/1
  Mux57/1 -> [Traffic_Info_05]
  Mux46/1 -> [Traffic_Info_20]
  Gain/1 -> Sum/2
  Bus Selector20/6 -> Mux40/6  "<a_0 y>"
  Constant15/1 -> Traffic Object9/1
  Bus Selector29/3 -> Mux60/3  "<r_zyx z>"
  [Traffic_Info_02] -> Mux59/3
  Constant111/1 -> MATLAB Function/5(goalIdx), MATLAB Function4 1/4(TRIGGER_IDX)
  Bus Selector9/1 -> Mux12/1  "<t_0 x>"
  Constant16/1 -> Mux11/1
  Constant77/1 -> Traffic Object6/1
  Mux15/1 -> Mux14/4
  Mux1/1 -> [Traffic_Info_01]
  Mux10/1 -> [Traffic_Info_07]
  Traffic Object15/2 -> Bus Selector15/1
  Constant62/1 -> Mux37/2
  Constant94/1 -> Mux61/2
  Constant57/1 -> Mux35/2
  Constant20/1 -> Traffic Object7/1
  Traffic Object30/1 -> Terminator30/1
  [Traffic_Info_06] -> Mux59/7
  Constant117/1 -> MATLAB Function/4(must2)
  MATLAB Function6/2(traffic_lane_idx) -> [traffic_lane_idx]
  Constant84/1 -> Traffic Object27/1
  [Traffic_Info_08] -> Mux59/9
  Bus Selector31/3 -> Mux64/3  "<v_0 x>"
  Constant17/1 -> Mux11/2
  Mux58/1 -> Mux57/4
  Bus Selector7/3 -> Mux10/3  "<r_zyx z>"
  [Traffic_Info_07] -> Mux59/8
  Bus Selector14/3 -> Mux30/3  "<r_zyx z>"
  Bus Selector15/1 -> Mux28/1  "<t_0 x>"
  From9/1 -> PID for parking/1
  Constant14/1 -> Mux58/2
  MATLAB Function4 1/1(G2P) -> [flag_to_G2P]
  Constant43/1 -> Mux27/2
  [Traffic_Info_16] -> Mux59/17
  [Ego_Gloabl_Y] -> Mux3/2
  Bus Selector21/2 -> Mux42/2  "<t_0 y>"
  Bus Selector21/3 -> Mux42/3  "<v_0 x>"
  MATLAB Function3/1(lateral_error) -> [LateralError]
  Bus Selector13/2 -> Mux26/2  "<t_0 y>"
  [Traffic_Info_03] -> Mux59/4
  Constant51/1 -> Traffic Object17/1
  Transpose8/1 -> Matrix Concatenate2/1
  Traffic Object28/2 -> Bus Selector31/1
  Traffic Object4/2 -> Bus Selector3/1
  Bus Selector26/1 -> Mux54/1  "<t_0 x>"
  Constant60/1 -> Traffic Object16/1
  Read CM Dict24/1 -> Mux44/8
  Read CM Dict8/1 -> [Ego_Yaw]
  Constant50/1 -> Mux31/2
  Traffic Object13/1 -> Terminator13/1
  [Traffic_Info_23] -> Transpose10/1
  Bus Selector11/3 -> Mux20/3  "<r_zyx z>"
  Bus Selector25/5 -> Mux50/5  "<a_0 x>"
  Mux18/1 -> [Traffic_Info_11]
  Constant97/1 -> Mux65/2
  [Global_Waypoints4] -> MATLAB Function4 1/1(global_waypoints_in)
  Traffic Object9/1 -> Terminator9/1
  [Global_Waypoints3] -> MATLAB Function6/5(wp3)
  [Traffic_Info_14] -> Mux59/15
  Traffic Object26/2 -> Bus Selector25/1
  [Ego_Global_X] -> MATLAB Function4 1/2(x_ego)
  Constant96/1 -> Mux65/1
  Mux59/1 -> Traffic_Info/1
  Bus Selector10/1 -> Mux22/1  "<t_0 x>"
  Mux35/1 -> Mux34/4
  Mux5/1 -> [Traffic_Info_02]
  PID for parking/1 -> Sum1/2
  Mux47/1 -> Mux46/4
  [Ego_Velocity] -> Add/2
  Bus Selector26/3 -> Mux54/3  "<v_0 x>"
  Bus Selector14/2 -> Mux30/2  "<t_0 y>"
  [Global_Waypoints1] -> MATLAB Function6/3(wp1)
  Constant88/1 -> Mux56/1
  Bus Selector13/1 -> Mux26/1  "<t_0 x>"
  Bus Selector19/2 -> Mux36/2  "<t_0 y>"
  Traffic Object17/2 -> Bus Selector16/1
  Mux9/1 -> [Traffic_Info_03]
  Bus Selector15/2 -> Mux28/2  "<t_0 y>"
  Bus Selector23/6 -> Mux44/6  "<a_0 y>"
  [Traffic_Info_28] -> Mux59/29
  Bus Selector9/3 -> Mux12/3  "<r_zyx z>"
  Constant25/1 -> Traffic Object31/1
  Mux4/1 -> Mux1/4
  Traffic Object29/1 -> Terminator29/1
  Constant56/1 -> Mux35/1
  Saturation1/1 -> Write CM Dict4/1, Write CM Dict3/1
  Traffic Object12/1 -> Terminator12/1
  [Traffic_Info_13] -> Mux59/14
  Bus Selector31/5 -> Mux64/5  "<a_0 x>"
  [ego_lane_idx] -> MATLAB Function5/4(ego_lane_idx)
  Constant70/1 -> Mux43/2
  Constant55/1 -> Mux8/1
  Constant30/1 -> Mux19/2
  Constant92/1 -> Mux61/1
  Mux26/1 -> [Traffic_Info_15]
  Traffic Object14/2 -> Bus Selector13/1
  Constant83/1 -> Mux51/2
  Constant33/1 -> Mux4/2
  Traffic Object6/1 -> ?
  Constant47/1 -> Traffic Object12/1
  Bus Selector25/4 -> Mux50/4  "<v_0 y>"
  Bus Selector11/2 -> Mux20/2  "<t_0 y>"
  Bus Selector17/2 -> Mux34/2  "<t_0 y>"
  Bus Selector21/7 -> Mux42/7  "<r_zyx z>"
  Constant91/1 -> Traffic Object3/1
  Bus Selector8/2 -> Mux14/2  "<t_0 y>"
  Constant48/1 -> Mux31/1
  Constant32/1 -> Mux21/1
  [New_Waypoint] -> "MATLAB Function4 "/1(waypoints)
  Constant12/1 -> Traffic Object8/1
  [Target_speed2] -> MATLAB Function1/4(target_speed_in)
  Constant71/1 -> Traffic Object23/1
  [Local_Points] -> MATLAB Function4/1(local_waypoints)
  Bus Selector24/5 -> Mux48/5  "<a_0 x>"
  Bus Selector24/3 -> Mux48/3  "<v_0 x>"
  Traffic Object19/1 -> Terminator19/1
  Constant78/1 -> Traffic Object25/1
  Rate Limiter1/1 -> [Target_speed2]
  Traffic Object29/2 -> Bus Selector9/1
  Sum/1 -> Saturation1/1
  [Ego_Gloabl_Y] -> Mux/2
  Traffic Object27/2 -> Bus Selector27/1
  [Traffic_Info_21] -> Transpose8/1
  Bus Selector4/2 -> Mux5/2  "<t_0 y>"
  Bus Selector23/2 -> Mux44/2  "<t_0 y>"
  Traffic Object6/2 -> Bus Selector5/1
  Traffic Object5/2 -> Bus Selector4/1
  Mux42/1 -> [Traffic_Info_22]
  Constant9/1 -> [Global_Waypoints3]
  [Global_Waypoints2] -> MATLAB Function6/4(wp2)
  Bus Selector3/3 -> Mux1/3  "<r_zyx z>"
  Mux22/1 -> [Traffic_Info_09]
  Add/1 -> PID Controller1/1
  Mux64/1 -> [Traffic_Info_28]
  Bus Selector25/6 -> Mux50/6  "<a_0 y>"
  Bus Selector27/7 -> Mux52/7  "<r_zyx z>"
  [Ego_Gloabl_Y] -> MATLAB Function4 1/3(y_ego)
  [Traffic_Info_18] -> Mux59/19
  [Traffic_Info_25] -> Transpose12/1
  Constant76/1 -> Mux47/2
  Mux14/1 -> [Traffic_Info_04]
  Traffic Object13/2 -> Bus Selector12/1
  Traffic Object22/1 -> Terminator22/1
  Constant26/1 -> Mux17/1
  Bus Selector27/6 -> Mux52/6  "<a_0 y>"
  [Ego_Yaw] -> MATLAB Function5/2(ego_yaw)
  Bus Selector16/3 -> Mux32/3  "<r_zyx z>"
  Constant65/1 -> Mux41/1
  Traffic Object10/1 -> Terminator10/1
  Traffic Object21/2 -> Bus Selector20/1
  Mux40/1 -> [Traffic_Info_21]
  Constant64/1 -> Traffic Object21/1
  Constant42/1 -> Mux27/1
  Bus Selector6/3 -> Mux57/3  "<r_zyx z>"
  Constant45/1 -> Traffic Object15/1
  Constant19/1 -> Mux13/1
  Bus Selector22/1 -> Mux46/1  "<t_0 x>"
  Traffic Object8/2 -> Bus Selector6/1
  Transpose12/1 -> Matrix Concatenate2/5
  [onRoad_Traffic] -> MATLAB Function5/5(traffic_info), MATLAB Function6/2(traffic_info)
  Bus Selector28/2 -> Mux16/2  "<t_0 y>"
  [Ego_Velocity] -> MATLAB Function5/3(ego_vx)
  Bus Selector16/1 -> Mux32/1  "<t_0 x>"
  Mux45/1 -> Mux44/9
  Constant36/1 -> Mux21/2
  Mux37/1 -> Mux36/4
  MATLAB Function/1(global_path_xy_dense) -> To Workspace/1, [New_Waypoint]
  Matrix Concatenate2/1 -> [onRoad_Traffic]
  Bus Selector8/1 -> Mux14/1  "<t_0 x>"
  [Traffic_Info_21] -> Mux59/22
  Bus Selector25/3 -> Mux50/3  "<v_0 x>"
  Constant22/1 -> Mux4/1
  Bus Selector24/6 -> Mux48/6  "<a_0 y>"
  [Traffic_Info_26] -> Transpose13/1
  Bus Selector26/2 -> Mux54/2  "<t_0 y>"
  Traffic Object4/1 -> ?
  Bus Selector10/2 -> Mux22/2  "<t_0 y>"
  Bus Selector17/1 -> Mux34/1  "<t_0 x>"
  Bus Selector31/2 -> Mux64/2  "<t_0 y>"
  Constant80/1 -> Mux49/2
  Traffic Object15/1 -> Terminator15/1
  Traffic Object31/2 -> Bus Selector28/1
  Constant11/1 -> Traffic Object4/1
  Bus Selector25/1 -> Mux50/1  "<t_0 x>"
  Gain1/1 -> Sum1/1
  Bus Selector5/3 -> Mux9/3  "<r_zyx z>"
  Mux50/1 -> [Traffic_Info_26]
  Constant44/1 -> Traffic Object5/1
  Constant67/1 -> Mux41/2
  Traffic Object26/1 -> Terminator26/1
  Bus Selector6/1 -> Mux57/1  "<t_0 x>"
  [Ego_Global_X] -> Mux/1
  [Ego_Global_X] -> MATLAB Function1/1(u1)
  Bus Selector20/1 -> Mux40/1  "<t_0 x>"
  Transpose10/1 -> Matrix Concatenate2/3
  Traffic Object20/1 -> Terminator20/1
  Bus Selector31/7 -> Mux64/7  "<r_zyx z>"
  Bus Selector23/5 -> Mux44/5  "<a_0 x>"
  Bus Selector24/2 -> Mux48/2  "<t_0 y>"
  Bus Selector20/4 -> Mux40/4  "<v_0 y>"
  Constant31/1 -> Traffic Object11/1
  Constant58/1 -> Traffic Object19/1
  Mux34/1 -> [Traffic_Info_19]
  Bus Selector27/1 -> Mux52/1  "<t_0 x>"
  Constant8/1 -> [Global_Waypoints2]
  Constant114/1 -> MATLAB Function/1(waypoints_in)
  Read CM Dict23/1 -> Mux42/8
  Constant41/1 -> Traffic Object14/1
  Mux36/1 -> [Traffic_Info_06]
  From58/1 -> Gain1/1
  [Traffic_Info_12] -> Mux59/13
  Mux51/1 -> Mux50/9
  Mux/1 -> "MATLAB Function4 "/2(vehicle_position)
  [Traffic_Info_00] -> Mux59/1
  Read CM Dict27/1 -> Mux50/8
  Transpose15/1 -> Matrix Concatenate2/8
  MATLAB Function5/2(debug_time_gap) -> Scope8/1
  Constant79/1 -> Mux49/1
  Constant63/1 -> Mux39/2
  Bus Selector23/3 -> Mux44/3  "<v_0 x>"
  Constant82/1 -> Mux51/1
  Constant7/1 -> MATLAB Function3/3(lookahead_time)
  Constant69/1 -> Mux43/1
  Bus Selector22/2 -> Mux46/2  "<t_0 y>"
  Traffic Object24/2 -> Bus Selector26/1
  Constant49/1 -> Mux29/2
  Traffic Object3/1 -> ?
  Constant13/1 -> Mux58/1
  Bus Selector21/1 -> Mux42/1  "<t_0 x>"
  PID Controller2/1 -> Write CM Dict6/1
  PID for parking1/1 -> Sum3/2
  Saturation2/1 -> Write CM Dict2/1, Write CM Dict1/1
  Rate Limiter/1 -> Goto45/1
  Mux2/1 -> MATLAB Function4 2/2(vehicle_position)
  Mux6/1 -> MATLAB Function10/1(ego_pos)
  Constant2/1 -> MATLAB Function2/1(waypoints)
  Constant4/1 -> MATLAB Function2/3(must1)
  From98/1 -> MATLAB Function11/3(ego_vx)
  From34/1 -> MATLAB Function4 3/1(global_waypoints)
  Gain3/1 -> Sum3/1
  MATLAB Function4 3/1(flag) -> Goto10/1
  Add1/1 -> PID Controller2/1
  From90/1 -> Mux62/2
  From64/1 -> Transpose4/1
  Transpose2/1 -> Matrix Concatenate/3
  From36/1 -> MATLAB Function10/3(wp1)
  From71/1 -> Transpose6/1
  From97/1 -> MATLAB Function7/1(u1)
  Constant1/1 -> MATLAB Function2/5(goalIdx)
  From96/1 -> MATLAB Function8/1(poly_coeff)
  Constant3/1 -> MATLAB Function2/2(startIdx)
  From48/1 -> Mux6/1
  From35/1 -> MATLAB Function4 2/3(head)
  From65/1 -> Transpose5/1
  From88/1 -> MATLAB Function4 2/1(waypoints)
  From56/1 -> Transpose2/1
  Matrix Concatenate/1 -> MATLAB Function10/2(traffic_info), MATLAB Function11/5(traffic_info)
  From91/1 -> MATLAB Function11/2(ego_yaw)
  From101/1 -> MATLAB Function8/2(velocity)
  From99/1 -> Transpose7/1
  MATLAB Function10/1(ego_lane_idx) -> Goto43/1
  MATLAB Function4 2/1(local_waypoints_) -> Goto7/1
  From86/1 -> MATLAB Function9/1(local_waypoints)
  Transpose6/1 -> Matrix Concatenate/7
  MATLAB Function9/1(poly_coeff) -> Goto8/1
  From53/1 -> Mux2/2
  From50/1 -> Mux2/1
  From52/1 -> Transpose1/1
  Transpose/1 -> Matrix Concatenate/1
  From87/1 -> MATLAB Function4 3/3(y_ego)
  From66/1 -> Add1/2
  Transpose3/1 -> Matrix Concatenate/4
  Gain2/1 -> Sum2/2
  MATLAB Function11/2(debug_dist) -> Scope1/1
  From51/1 -> Transpose/1
  Mux62/1 -> MATLAB Function11/1(ego_pos)
  MATLAB Function8/6(kappa) -> Goto6/1
  Transpose1/1 -> Matrix Concatenate/2
  MATLAB Function7/1(target_speed_out) -> Add1/1
  Constant10/1 -> MATLAB Function8/3(lookahead_time)
  MATLAB Function11/1(target_speed) -> Rate Limiter/1
  From63/1 -> Transpose3/1
  MATLAB Function8/1(lateral_error) -> Goto9/1
  Transpose5/1 -> Matrix Concatenate/6
  Transpose4/1 -> Matrix Concatenate/5
  Constant5/1 -> MATLAB Function2/4(must2)
  From49/1 -> Mux6/2
  From67/1 -> MATLAB Function7/3(target_speed_in)
  Sum3/1 -> Gain2/1
  Transpose7/1 -> Matrix Concatenate/8
  From89/1 -> Mux62/1
  From93/1 -> MATLAB Function11/6(traffic_lane_idx)
  From85/1 -> MATLAB Function4 3/2(x_ego)
  From72/1 -> Gain3/1
  MATLAB Function2/1(global_path_xy_dense) -> To Workspace1/1, Goto11/1
  From38/1 -> MATLAB Function10/5(wp3)
  From102/1 -> PID for parking1/1
  From37/1 -> MATLAB Function10/4(wp2)
  Sum2/1 -> Saturation2/1
  MATLAB Function10/2(traffic_lane_idx) -> Goto42/1
  From92/1 -> MATLAB Function11/4(ego_lane_idx)
  From100/1 -> MATLAB Function7/2(u2)
  Mux3/1 -> MATLAB Function6/1(ego_pos)
  Saturation3/1 -> Write CM Dict8/1, Write CM Dict7/1
  MATLAB Function12/1(steering_angle) -> Saturation3/1
  Constant/1 -> MATLAB Function12/1(waypoints)
  [Ego_Gloabl_Y] -> Mux63/2
  [Ego_Global_X] -> Mux63/1
  Mux63/1 -> MATLAB Function12/2(vehicle_position)
  [Ego_Yaw] -> MATLAB Function12/3(head)
  MATLAB Function1/2(finish_flag) -> [G2P_Finish]
  [G2P_Finish] -> Output1/1
  [Ego_Yaw] -> MATLAB Function1/3(u3)
